simulink model "sampleModel192"  (R2021b)
settings: Solver=VariableStepAuto  StartTime=0.0  StopTime=10.0  RelTol=1e-3
undefined symbols (not defined in the file or in its folder): DiscIntNeverNeededParam, Newton, Raphson
libraries: simulink x4
settings Model: Creator=user  LastModifiedBy=user

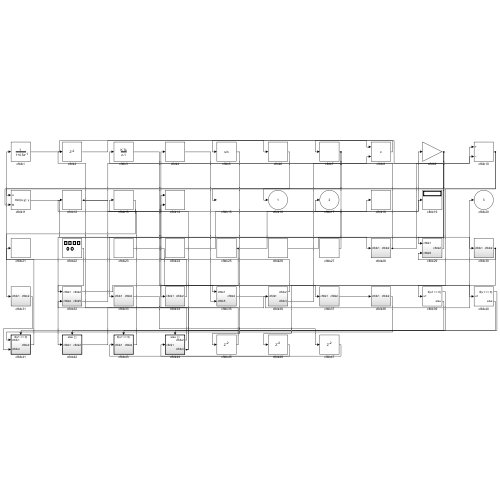
[thumbnail: Simulink's stored preview of the top-level diagram]
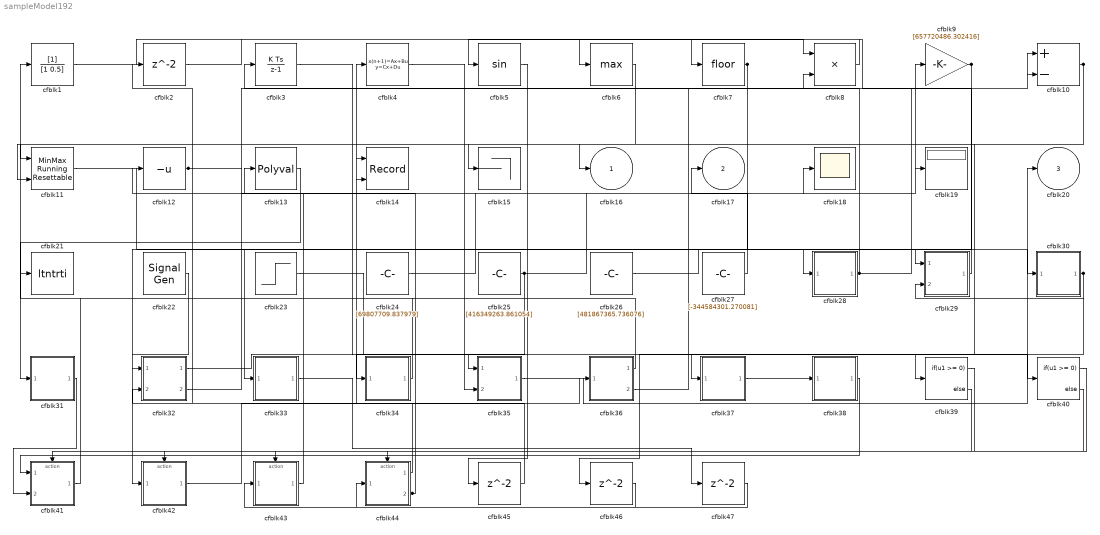
== system sampleModel192 ==
  cfblk1 : DiscreteFilter  SampleTime=1
  cfblk10 : Sum  Inputs=+-
  cfblk11 : simulink/Math Operations/MinMax Running Resettable  Function=min  vinit=0.0
  cfblk12 : UnaryMinus
  cfblk13 : Polyval  Coefs=[ +2.081618890e-019, -1.441693666e-014, +4.719686976e-010, -8.536869453e-006, +1.621573104e-001, -8.087801117e+001 ]
  cfblk14 : Record  FileSettingsInternal="{\"entries\":[{\"content\":{\"excelSettings\":{\"content\":{},\"type\":\"Streamout.ExcelSettings\"}},\"type\":\"Streamout.FileSettingStorage\",\"uuid\":\"9ac6d932-b654-4180-a5f7-901607cb5b3d\"}],\"packageUris\":[\"http://schema.mathworks.com/mf0/streamout_blocks/R2020a\"],\"version\":\"1.0\"}"  Layout=[1 1]  SignalsInternal="{\"entries\":[{\"content\":{\"signals\":[{\"content\":{\"blockPath\":[\"sampleModel192/cfblk14\"],\"channel\":[],\"dimensions\":[1],\"domain\":\"sampleModel192/cfblk14\",\"lineColor\":\"#a2142f\",\"plots\":[1],\"port\":1,\"sid\":[\"\"],\"signalID\":7173,\"signalName\":\"cfblk44:1\"},\"type\":\"RecordBlkView.Signal\",\"uuid\":\"3e7a05fb-5f3e-420c-8636-6d6213171b52\"},{\"content\":{\"blockPath\":[\"sampleModel192/cfblk14\"],\"channel\":[],\"dimensions\":[1],\"domain\":\"sampleModel192/cfblk14\",\"lineColor\":\"#139fff\",\"plots\":[1],\"port\":2,\"sid\":[\"\"],\"signalID\":7177,\"signalName\":\"cfblk12\"},\"type\":\"RecordBlkView.Signal\",\"uuid\":\"892913ae-0b6a-49d0-967f-99abf78f11db\"}]},\"type\":\"RecordBlkView.InputSignals\",\"uuid\":\"bcc50052-22dd-407c-9a3f-eca97caaa135\"}],\"packageUris\":[\"http://schema.mathworks.com/mf0/streamout_blocks/R2020a\"],\"version\":\"1.0\"}"  VisualizationBindings="{\"xyplotplugin\":{\"info\":[{\"series\":[{\"bindingParametersList\":[{\"parameter\":\"X-Axis\",\"signalID\":7173,\"signalName\":\"cfblk44:1\"},{\"parameter\":\"Y-Axis\",\"signalID\":7177,\"signalName\":\"cfblk12\"}],\"seriesID\":9250}],\"subplotID\":1}]}}"  CompatibilityTag=XY
  cfblk15 : Terminator
  cfblk18 : Scope
  cfblk19 : Display
  cfblk{2,45..47} (4 alike) : Delay  SampleTime=1
  cfblk21 : ToWorkspace  VariableName=ltntrti  SaveFormat=Timeseries  SampleTime=-1
  cfblk22 : SignalGenerator  WaveForm=square  Amplitude=[20018358.018870]  Units=rad/sec
  cfblk23 : Step  Time=[37.000000]  Before=[-261303681.661120]  After=[790231344.462122]  SampleTime=0
  cfblk24 : Constant  Value=[69807709.837979]  SampleTime=1
  cfblk25 : Constant  Value=[416349263.861054]  SampleTime=1
  cfblk26 : Constant  Value=[481867365.736076]  SampleTime=1
  cfblk27 : Constant  Value=[-344584301.270081]  SampleTime=1
  cfblk28 : Subsystem
  cfblk29 : Subsystem
  cfblk3 : DiscreteIntegrator  ICPrevOutput=DiscIntNeverNeededParam  ICPrevScaledInput=DiscIntNeverNeededParam
  cfblk30 : Subsystem
  cfblk31 : Subsystem
  cfblk32 : Subsystem
  cfblk33 : Subsystem
  cfblk34 : Subsystem
  cfblk35 : Subsystem
  cfblk36 : Subsystem
  cfblk37 : Subsystem
  cfblk38 : Subsystem
  cfblk39 : If  IfExpression=u1 >= 0  SampleTime=1
  cfblk4 : DiscreteStateSpace
  cfblk40 : If  IfExpression=u1 >= 0  SampleTime=1
  cfblk41 : Subsystem  TreatAsAtomicUnit=on
  cfblk42 : Subsystem  TreatAsAtomicUnit=on
  cfblk43 : Subsystem  TreatAsAtomicUnit=on
  cfblk44 : Subsystem  TreatAsAtomicUnit=on
  cfblk5 : Trigonometry
  cfblk6 : MinMax  Function=max
  cfblk7 : Rounding
  cfblk8 : Product  Inputs=**
  cfblk9 : Gain  Gain=[657720486.302416]
  cfblk16 : Outport
  cfblk17 : Outport  Port=2
  cfblk20 : Outport  Port=3
  wires:
  cfblk32/1(cfblk2) -> cfblk37/1(cfblk1)
  cfblk35/1(cfblk2) -> cfblk20/1
  cfblk28/1(cfblk2) -> cfblk3/1, cfblk10/2
  cfblk29/1(cfblk2) -> cfblk7/1
  cfblk30/1(cfblk2) -> cfblk29/2(cfblk5), cfblk46/1
  cfblk37/1(cfblk2) -> cfblk38/1(cfblk1)
  cfblk26/1 -> cfblk28/1(cfblk1)
  cfblk27/1 -> cfblk17/1
  cfblk7/1 -> cfblk33/1(cfblk1), cfblk15/1
  cfblk13/1 -> cfblk31/1(cfblk1)
  cfblk34/1(cfblk2) -> cfblk4/1
  cfblk8/1 -> cfblk5/1
  cfblk6/1 -> cfblk16/1
  cfblk25/1 -> cfblk9/1, cfblk34/1(cfblk1)
  cfblk36/1(cfblk2) -> cfblk1/1
  cfblk10/1 -> cfblk39/1, cfblk11/1
  cfblk32/2(cfblk5) -> cfblk18/1
  cfblk11/1 -> cfblk30/1(cfblk1)
  cfblk38/1(cfblk2) -> cfblk41/1(cfblk1)
  cfblk22/1 -> cfblk42/1(cfblk1)
  cfblk31/1(cfblk2) -> cfblk41/2(cfblk4)
  cfblk44/1(cfblk2) -> cfblk14/1
  cfblk43/1(cfblk2) -> cfblk13/1
  cfblk1/1 -> cfblk6/1
  cfblk9/1 -> cfblk29/1(cfblk1), cfblk32/1(cfblk1), cfblk11/2
  cfblk41/1(cfblk2) -> cfblk21/1
  cfblk44/2(cfblk4) -> cfblk12/1, cfblk32/2(cfblk4)
  cfblk24/1 -> cfblk19/1
  cfblk4/1 -> cfblk40/1
  cfblk42/1(cfblk2) -> cfblk36/1(cfblk1)
  cfblk3/1 -> cfblk35/1(cfblk1)
  cfblk2/1 -> cfblk8/1
  cfblk12/1 -> cfblk14/2, cfblk10/1
  cfblk23/1 -> cfblk35/2(cfblk5)
  cfblk36/2(cfblk3) -> cfblk8/2
  cfblk39/1 -> cfblk41/Action
  cfblk39/2 -> cfblk42/Action
  cfblk40/1 -> cfblk43/Action
  cfblk40/2 -> cfblk44/Action
  cfblk5/1 -> cfblk45/1
  cfblk45/1 -> cfblk2/1
  cfblk46/1 -> cfblk43/1(cfblk1)
  cfblk33/1(cfblk2) -> cfblk47/1
  cfblk47/1 -> cfblk44/1(cfblk1)

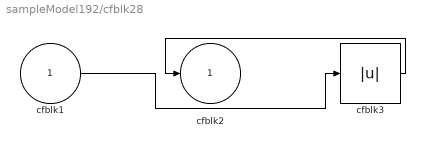
== system sampleModel192/cfblk28 ==
  cfblk1 : Inport
  cfblk3 : Abs
  cfblk2 : Outport
  wires:
  cfblk3/1 -> cfblk2/1
  cfblk1/1 -> cfblk3/1

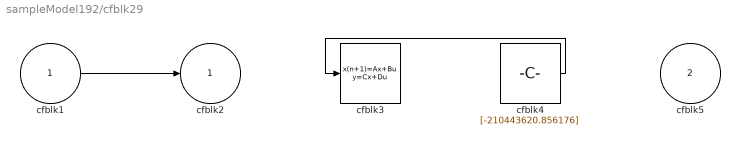
== system sampleModel192/cfblk29 ==
  cfblk1 : Inport
  cfblk5 : Inport  Port=2
  cfblk3 : DiscreteStateSpace
  cfblk4 : Constant  Value=[-210443620.856176]  SampleTime=1
  cfblk2 : Outport
  wires:
  cfblk4/1 -> cfblk3/1
  cfblk1/1 -> cfblk2/1

== system sampleModel192/cfblk30 ==
  cfblk1 : Inport
  cfblk3 : simulink/Discrete/Transfer Fcn First Order  PoleZ=0.95  ICPrevOutput=0.0  DoSatur=off
  cfblk2 : Outport
  wires:
  cfblk1/1 -> cfblk2/1, cfblk3/1

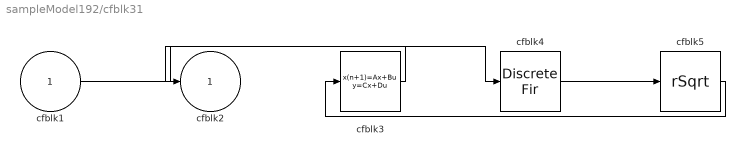
== system sampleModel192/cfblk31 ==
  cfblk1 : Inport
  cfblk3 : DiscreteStateSpace
  cfblk4 : DiscreteFir  SampleTime=1
  cfblk5 : Sqrt  Operator=rSqrt  AlgorithmType=Newton-Raphson  SaturateOnIntegerOverflow=on
  cfblk2 : Outport
  wires:
  cfblk4/1 -> cfblk5/1
  cfblk1/1 -> cfblk4/1
  cfblk5/1 -> cfblk3/1
  cfblk3/1 -> cfblk2/1

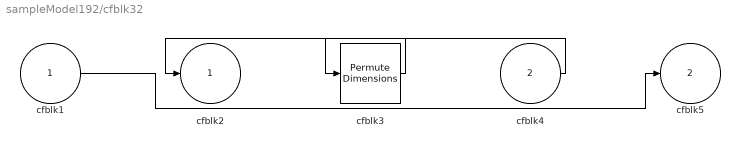
== system sampleModel192/cfblk32 ==
  cfblk1 : Inport
  cfblk4 : Inport  Port=2
  cfblk3 : PermuteDimensions
  cfblk2 : Outport
  cfblk5 : Outport  Port=2
  wires:
  cfblk3/1 -> cfblk2/1
  cfblk1/1 -> cfblk5/1
  cfblk4/1 -> cfblk3/1

== system sampleModel192/cfblk33 ==
  cfblk1 : Inport
  cfblk3 : Constant  Value=[542634719.257222]  SampleTime=1
  cfblk2 : Outport
  wires:
  cfblk1/1 -> cfblk2/1

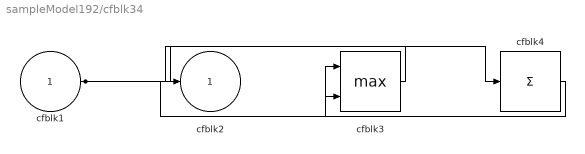
== system sampleModel192/cfblk34 ==
  cfblk1 : Inport
  cfblk3 : MinMax  Function=max  Inputs=2
  cfblk4 : Sum  Inputs=+
  cfblk2 : Outport
  wires:
  cfblk1/1 -> cfblk4/1, cfblk3/2
  cfblk4/1 -> cfblk3/1
  cfblk3/1 -> cfblk2/1

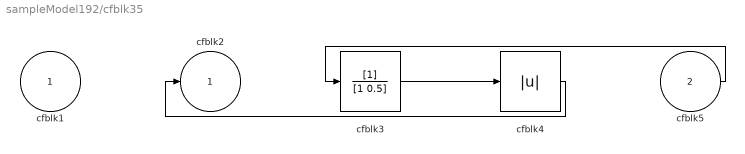
== system sampleModel192/cfblk35 ==
  cfblk1 : Inport
  cfblk5 : Inport  Port=2
  cfblk3 : DiscreteFilter  SampleTime=1
  cfblk4 : Abs
  cfblk2 : Outport
  wires:
  cfblk5/1 -> cfblk3/1
  cfblk3/1 -> cfblk4/1
  cfblk4/1 -> cfblk2/1

== system sampleModel192/cfblk36 ==
  cfblk1 : Inport
  cfblk2 : Outport
  cfblk3 : Outport  Port=2
  wires:
  cfblk1/1 -> cfblk3/1, cfblk2/1

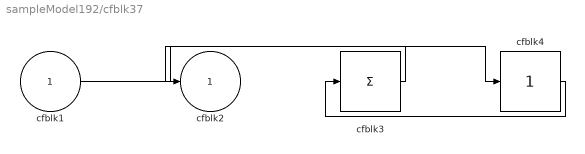
== system sampleModel192/cfblk37 ==
  cfblk1 : Inport
  cfblk3 : Sum  Inputs=+
  cfblk4 : simulink/Math Operations/Slider Gain  gain=1  low=0  high=2
  cfblk2 : Outport
  wires:
  cfblk1/1 -> cfblk4/1
  cfblk4/1 -> cfblk3/1
  cfblk3/1 -> cfblk2/1

== system sampleModel192/cfblk38 ==
  cfblk1 : Inport
  cfblk3 : simulink/Discrete/Transfer Fcn First Order  PoleZ=0.95  ICPrevOutput=0.0  DoSatur=off
  cfblk2 : Outport
  wires:
  cfblk3/1 -> cfblk2/1
  cfblk1/1 -> cfblk3/1

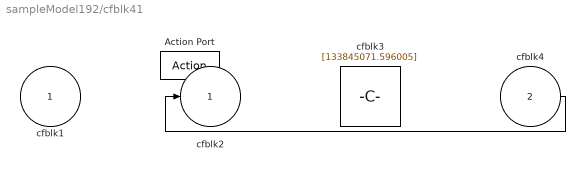
== system sampleModel192/cfblk41 ==
  cfblk1 : Inport
  cfblk4 : Inport  Port=2
  Action Port : ActionPort  ActionPortLabel=if(u1 >= 0)
  cfblk3 : Constant  Value=[133845071.596005]  SampleTime=1
  cfblk2 : Outport
  wires:
  cfblk4/1 -> cfblk2/1

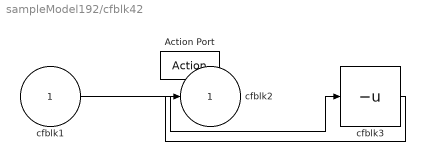
== system sampleModel192/cfblk42 ==
  cfblk1 : Inport
  Action Port : ActionPort  ActionPortLabel=else
  cfblk3 : UnaryMinus
  cfblk2 : Outport
  wires:
  cfblk1/1 -> cfblk3/1
  cfblk3/1 -> cfblk2/1

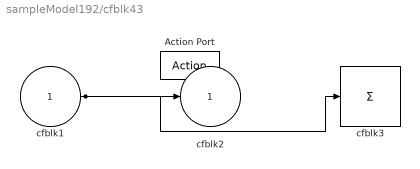
== system sampleModel192/cfblk43 ==
  cfblk1 : Inport
  Action Port : ActionPort  ActionPortLabel=if(u1 >= 0)
  cfblk3 : Sum  Inputs=+
  cfblk2 : Outport
  wires:
  cfblk1/1 -> cfblk2/1, cfblk3/1

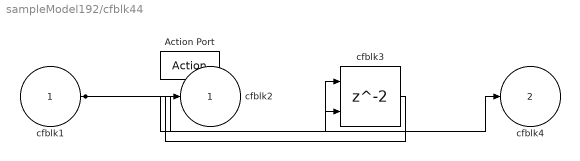
== system sampleModel192/cfblk44 ==
  cfblk1 : Inport
  Action Port : ActionPort  ActionPortLabel=else
  cfblk3 : Delay  ShowEnablePort=on
      settings: InputPortMap=u0,e6
  cfblk2 : Outport
  cfblk4 : Outport  Port=2
  wires:
  cfblk1/1 -> cfblk3/1, cfblk3/2, cfblk4/1
  cfblk3/1 -> cfblk2/1
